simulink model "task_2_scheme"  (R2024a)
settings: Solver=VariableStepAuto  StartTime=0.0  StopTime=50.0  RelTol=1e-3
libraries: simulink x2
settings Model: Creator=alexe  LastModifiedBy=alexe

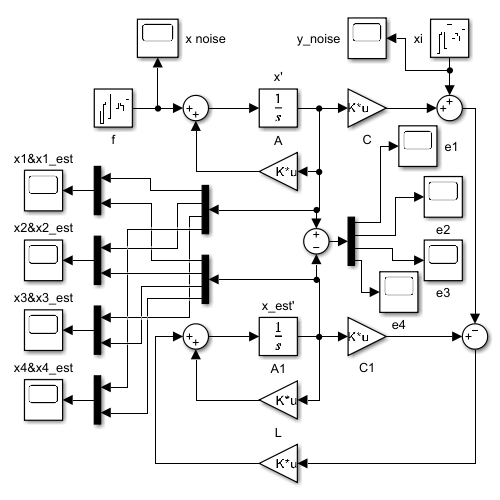
[thumbnail: Simulink's stored preview of the top-level diagram]
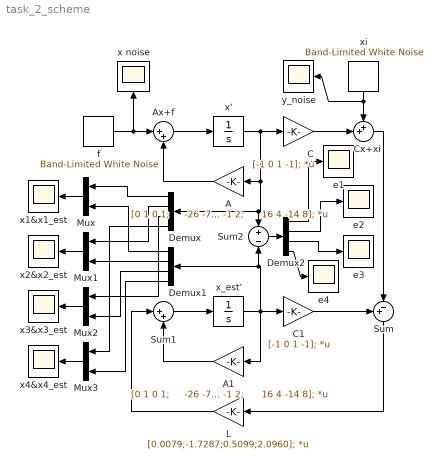
== system task_2_scheme ==
  A : Gain  Gain=|  Multiplication=Matrix(K*u)
      | [0 1 0 1;
      |     -26 -7 20 -11;
      |      0 1 -1 2;
      |      16 4 -14 8];
  A1 : Gain  Gain=|  Multiplication=Matrix(K*u)
      | [0 1 0 1;
      |     -26 -7 20 -11;
      |      0 1 -1 2;
      |      16 4 -14 8];
  Ax+f : Sum  Inputs=|++
  C : Gain  Gain=[-1 0 1 -1];  Multiplication=Matrix(K*u)
  C1 : Gain  Gain=[-1 0 1 -1];  Multiplication=Matrix(K*u)
  Cx+xi : Sum  Inputs=++|
  Demux : Demux
  Demux1 : Demux
  Demux2 : Demux
  L : Gain  Gain=[0.0079;-1.7287;0.5099;2.0960];  Multiplication=Matrix(K*u)
  Mux{,1..3} (4 alike) : Mux  Inputs=2
  Sum : Sum  Inputs=+-|
  Sum1 : Sum  Inputs=|++
  Sum2 : Sum  Inputs=+|-
  e{1..4} (4 alike) : Scope
  f : simulink/Sources/Band-Limited White Noise  Cov=[0.5]  Ts=1e-4  seed=[23341]  VectorParams1D=off
  x noise : Scope
  x' : Integrator  InitialCondition=[1;1;1;1];
  x1&x1_est : Scope
  x2&x2_est : Scope
  x3&x3_est : Scope
  x4&x4_est : Scope
  x_est' : Integrator  InitialCondition=[0;0;0;0];
  xi : simulink/Sources/Band-Limited White Noise  Cov=[1]  Ts=1e-4  seed=[23341]  VectorParams1D=off
  y_noise : Scope
  wires:
  A/1 -> Ax+f/2
  x'/1 -> Demux/1, Sum2/1, A/1, C/1
  Ax+f/1 -> x'/1
  C/1 -> Cx+xi/2
  f/1 -> x noise/1, Ax+f/1
  xi/1 -> y_noise/1, Cx+xi/1
  x_est'/1 -> Demux1/1, Sum2/2, A1/1, C1/1
  C1/1 -> Sum/1
  Cx+xi/1 -> Sum/2
  Sum/1 -> L/1
  A1/1 -> Sum1/2
  Sum1/1 -> x_est'/1
  L/1 -> Sum1/1
  Mux/1 -> x1&x1_est/1
  Demux/1 -> Mux/1
  Demux1/1 -> Mux/2
  Mux1/1 -> x2&x2_est/1
  Demux/2 -> Mux1/1
  Demux1/2 -> Mux1/2
  Mux2/1 -> x3&x3_est/1
  Demux/3 -> Mux2/1
  Demux1/3 -> Mux2/2
  Mux3/1 -> x4&x4_est/1
  Demux/4 -> Mux3/1
  Demux1/4 -> Mux3/2
  Sum2/1 -> Demux2/1
  Demux2/1 -> e1/1
  Demux2/2 -> e2/1
  Demux2/3 -> e3/1
  Demux2/4 -> e4/1
